simulink model "TestingDynamics"  (R2019b)
settings: Solver=VariableStepAuto  StartTime=0.0  StopTime=10.0  RelTol=1e-3
values from neighbouring files (symbols this model uses):
  M_inv = inv(M_motor)    [HW7_v2_matlab.m]
  M_motor = [1, 1, 1, -1;             1, 1, -1, 1;             1, -1, -1, -1;             1, -1, 1, 1 ]    [HW7_v2_matlab.m]
  measurement_noise = 0.1    [kalman_matrices_calculator.m]
  tau2 = eval(max(solve(1/sqrt((tau2*2*pi*10)^2+1^2) == 1/sqrt(2), tau2)))    [HW7_v2_matlab.m]    (also in kalman_matrices_calculator.m = 0.0159154943092)
  V = 5    [HW7_v2_matlab.m]
  V0 = 5    [HW7_v2_matlab.m]
undefined symbols (not defined in the file or in its folder): A, Aaileron, Aelevator, Arudder, Athrust, B, Baileron, Belevator, Brudder, Bthrust, C, C_P, C_rollpitch, C_T, C_yaw, Caileron, Celevator, Crudder, Cthrust, D, Daileron, Delevator, Drudder, Dthrust, g, J, Jinv, Prop_H, Thrust_Sum, trim_state, UAV_mass
libraries: vrlib x3, simulink x2, dspmtrx3 x1
settings Model: Creator=cwhipp  LastModifiedBy=cwhipp

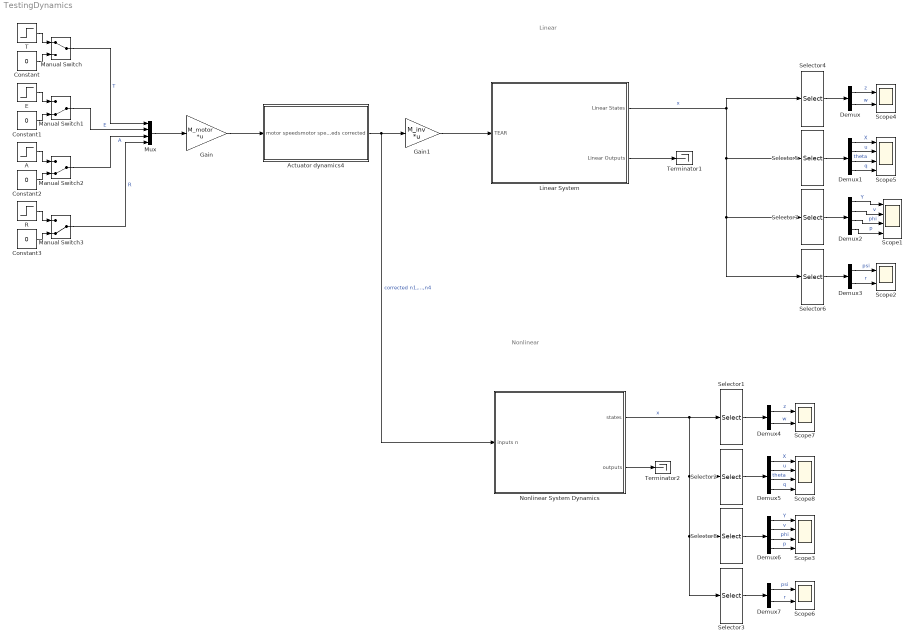
== system TestingDynamics ==
  note: Linear
  note: Nonlinear
  A : Step  SampleTime=0
  Actuator dynamics4 : Subsystem
  Constant{,1..3} (4 alike) : Constant  Value=0
  Demux{,3..4,7} (4 alike) : Demux  Outputs=2
  Demux{1..2,5..6} (4 alike) : Demux
  E : Step  SampleTime=0
  Gain : Gain  Gain=M_motor  Multiplication=Matrix(K*u)
  Gain1 : Gain  Gain=M_inv  Multiplication=Matrix(K*u)
  Linear System : Subsystem
  Manual Switch : ManualSwitch
  Manual Switch1 : ManualSwitch  CurrentSetting=0
  Manual Switch2 : ManualSwitch  CurrentSetting=0
  Manual Switch3 : ManualSwitch  CurrentSetting=0
  Mux : Mux
  Nonlinear System Dynamics : Subsystem
  R : Step  SampleTime=0
  Scope{1,3,5,8} (4 alike) : Scope  NumInputPorts=4
  Scope{2,4,6..7} (4 alike) : Scope  NumInputPorts=2
  Selector1 : Selector  InputPortWidth=12  IndexOptions=Index vector (dialog)  Indices=[3 6]  OutputSizes=1
  Selector2 : Selector  InputPortWidth=12  IndexOptions=Index vector (dialog)  Indices=[1 4 8 11]  OutputSizes=1
  Selector3 : Selector  InputPortWidth=12  IndexOptions=Index vector (dialog)  Indices=[9 12]  OutputSizes=1
  Selector4 : Selector  InputPortWidth=12  IndexOptions=Index vector (dialog)  Indices=[1 2]  OutputSizes=1
  Selector5 : Selector  InputPortWidth=12  IndexOptions=Index vector (dialog)  Indices=[3 4 5 6]  OutputSizes=1
  Selector6 : Selector  InputPortWidth=12  IndexOptions=Index vector (dialog)  Indices=[11 12]  OutputSizes=1
  Selector7 : Selector  InputPortWidth=12  IndexOptions=Index vector (dialog)  Indices=[7 8 9 10]  OutputSizes=1
  Selector8 : Selector  InputPortWidth=12  IndexOptions=Index vector (dialog)  Indices=[2 5 7 10]  OutputSizes=1
  T : Step  SampleTime=0
  Terminator1 : Terminator
  Terminator2 : Terminator
  wires:
  Linear System/1(Linear States) -> Selector4/1, Selector6/1, Selector7/1, Selector5/1  "x"
  Linear System/2(Linear Outputs) -> Terminator1/1
  Demux/2 -> Scope4/2  "w"
  Demux/1 -> Scope4/1  "z"
  Selector4/1 -> Demux/1
  Selector5/1 -> Demux1/1
  Demux1/1 -> Scope5/1  "X"
  Demux1/2 -> Scope5/2  "u"
  Demux1/3 -> Scope5/3  "theta"
  Demux1/4 -> Scope5/4  "q"
  T/1 -> Manual Switch/1
  Constant/1 -> Manual Switch/2
  E/1 -> Manual Switch1/1
  Constant1/1 -> Manual Switch1/2
  A/1 -> Manual Switch2/1
  Constant2/1 -> Manual Switch2/2
  R/1 -> Manual Switch3/1
  Constant3/1 -> Manual Switch3/2
  Manual Switch/1 -> Mux/1  "T"
  Manual Switch1/1 -> Mux/2  "E"
  Manual Switch2/1 -> Mux/3  "A"
  Manual Switch3/1 -> Mux/4  "R"
  Demux2/4 -> Scope1/4  "p"
  Demux2/1 -> Scope1/1  "Y"
  Selector7/1 -> Demux2/1
  Demux2/3 -> Scope1/3  "phi"
  Demux2/2 -> Scope1/2  "v"
  Demux3/2 -> Scope2/2  "r"
  Demux3/1 -> Scope2/1  "psi"
  Selector6/1 -> Demux3/1
  Gain/1 -> Actuator dynamics4/1(motor speeds)
  Mux/1 -> Gain/1
  Actuator dynamics4/1(motor speeds corrected) -> Nonlinear System Dynamics/1(inputs n), Gain1/1  "corrected n1,...,n4"
  Gain1/1 -> Linear System/1("TEAR ")
  Selector8/1 -> Demux6/1
  Demux7/2 -> Scope6/2  "r"
  Demux5/1 -> Scope8/1  "X"
  Nonlinear System Dynamics/1(states) -> Selector3/1, Selector8/1, Selector2/1, Selector1/1  "x"
  Demux5/4 -> Scope8/4  "q"
  Demux6/4 -> Scope3/4  "p"
  Selector1/1 -> Demux4/1
  Demux4/2 -> Scope7/2  "w"
  Demux4/1 -> Scope7/1  "z"
  Selector2/1 -> Demux5/1
  Demux6/1 -> Scope3/1  "Y"
  Demux6/3 -> Scope3/3  "phi"
  Selector3/1 -> Demux7/1
  Demux5/3 -> Scope8/3  "theta"
  Demux5/2 -> Scope8/2  "u"
  Demux7/1 -> Scope6/1  "psi"
  Demux6/2 -> Scope3/2  "v"
  Nonlinear System Dynamics/2(outputs) -> Terminator2/1

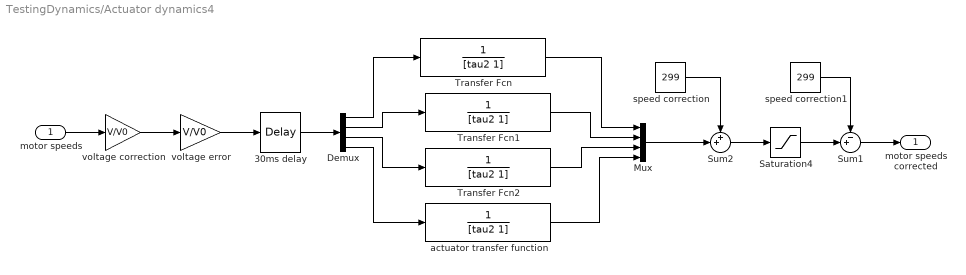
== system TestingDynamics/Actuator dynamics4 ==
  motor speeds : Inport
  30ms delay : TransportDelay  DelayTime=30e-3
  Demux : Demux
  Mux : Mux
  Saturation4 : Saturate  UpperLimit=500  LowerLimit=10
  Sum1 : Sum  Inputs=-+|
  Sum2 : Sum  Inputs=++|
  Transfer Fcn : TransferFcn  Denominator=[tau2 1]
  Transfer Fcn1 : TransferFcn  Denominator=[tau2 1]
  Transfer Fcn2 : TransferFcn  Denominator=[tau2 1]
  actuator transfer function : TransferFcn  Denominator=[tau2 1]
  speed correction : Constant  Value=299
  speed correction1 : Constant  Value=299
  voltage correction : Gain  Gain=V/V0
  voltage error : Gain  Gain=V/V0
  motor speeds corrected : Outport
  wires:
  speed correction/1 -> Sum2/1
  voltage correction/1 -> voltage error/1
  Sum2/1 -> Saturation4/1
  Demux/2 -> Transfer Fcn1/1
  30ms delay/1 -> Demux/1
  Demux/4 -> actuator transfer function/1
  Demux/1 -> Transfer Fcn/1
  Demux/3 -> Transfer Fcn2/1
  voltage error/1 -> 30ms delay/1
  motor speeds/1 -> voltage correction/1
  Transfer Fcn/1 -> Mux/1
  Transfer Fcn1/1 -> Mux/2
  Transfer Fcn2/1 -> Mux/3
  actuator transfer function/1 -> Mux/4
  Mux/1 -> Sum2/2
  Saturation4/1 -> Sum1/2
  Sum1/1 -> motor speeds corrected/1
  speed correction1/1 -> Sum1/1

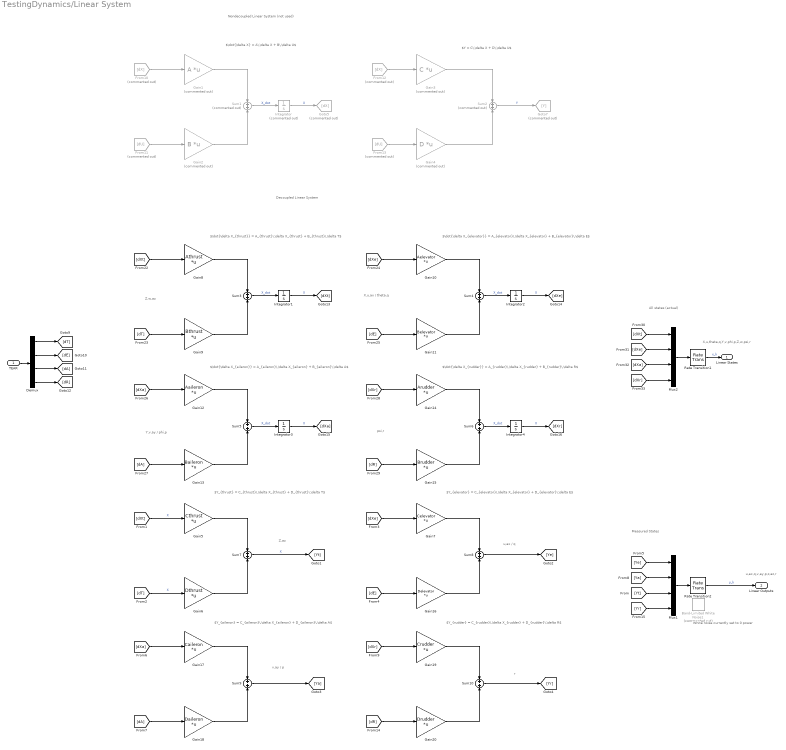
== system TestingDynamics/Linear System ==
  note: psi,r
  note: Y,v,ay / phi,p
  note: X,u,ax / theta,q
  note: Z,w,az
  note: Decoupled Linear System
  note: $\dot{\delta X} = A\,\delta X + B\,\delta U$
  note: $Y = C\,\delta X + D\,\delta U$
  note: $\dot{\delta X_{thrust}} = A_{thrust}\,\delta X_{thrust} + B_{thrust}\,\delta T$
  note: $\dot{\delta X_{elevator}} = A_{elevator}\,\delta X_{elevator} + B_{elevator}\,\delta E$
  note: $\dot{\delta X_{aileron}} = A_{aileron}\,\delta X_{aileron} + B_{aileron}\,\delta A$
  note: $\dot{\delta X_{rudder}} = A_{rudder}\,\delta X_{rudder} + B_{rudder}\,\delta R$
  note: Z,az
  note: u,ax / q
  note: v,ay / p
  note: r
  note: $Y_{thrust} = C_{thrust}\,\delta X_{thrust} + D_{thrust}\,\delta T$
  note: $Y_{elevator} = C_{elevator}\,\delta X_{elevator} + D_{elevator}\,\delta E$
  note: $Y_{aileron} = C_{aileron}\,\delta X_{aileron} + D_{aileron}\,\delta A$
  note: $Y_{rudder} = C_{rudder}\,\delta X_{rudder} + D_{rudder}\,\delta R$
  note: Nondecoupled Linear System (not used)
  note: All states (actual)
  note: Measured States
  note: u,ax,q,v,ay,p,z,az,r
  note: X,u,theta,q,Y,v,phi,p,Z,w,psi,r
  note: White noise currently set to 0 power
  "TEAR " : Inport
  Band-Limited White Noise1 : simulink/Sources/Band-Limited White Noise  Commented=on  Cov=measurement_noise*ones(9,1)*0  Ts=0.05  seed=[11;12;13;14;15;16;17;18;19]
  Demux : Demux
  From10 : From  Commented=on  GotoTag=dX
  From11 : From  Commented=on  GotoTag=dU
  From12 : From  Commented=on  GotoTag=dX
  From13 : From  Commented=on  GotoTag=dU
  Gain1 : Gain  Commented=on  Gain=A  Multiplication=Matrix(K*u)
  Gain10 : Gain  Gain=Aelevator  Multiplication=Matrix(K*u)
  Gain11 : Gain  Gain=Belevator  Multiplication=Matrix(K*u)
  Gain12 : Gain  Gain=Aaileron  Multiplication=Matrix(K*u)
  Gain13 : Gain  Gain=Baileron  Multiplication=Matrix(K*u)
  Gain14 : Gain  Gain=Arudder  Multiplication=Matrix(K*u)
  Gain15 : Gain  Gain=Brudder  Multiplication=Matrix(K*u)
  Gain16 : Gain  Gain=Delevator  Multiplication=Matrix(K*u)
  Gain17 : Gain  Gain=Caileron  Multiplication=Matrix(K*u)
  Gain18 : Gain  Gain=Daileron  Multiplication=Matrix(K*u)
  Gain19 : Gain  Gain=Crudder  Multiplication=Matrix(K*u)
  Gain2 : Gain  Commented=on  Gain=B  Multiplication=Matrix(K*u)
  Gain20 : Gain  Gain=Drudder  Multiplication=Matrix(K*u)
  Gain3 : Gain  Commented=on  Gain=C  Multiplication=Matrix(K*u)
  Gain4 : Gain  Commented=on  Gain=D  Multiplication=Matrix(K*u)
  Gain5 : Gain  Gain=Cthrust  Multiplication=Matrix(K*u)
  Gain6 : Gain  Gain=Dthrust  Multiplication=Matrix(K*u)
  Gain7 : Gain  Gain=Celevator  Multiplication=Matrix(K*u)
  Gain8 : Gain  Gain=Athrust  Multiplication=Matrix(K*u)
  Gain9 : Gain  Gain=Bthrust  Multiplication=Matrix(K*u)
  Goto5 : Goto  Commented=on  GotoTag=dX
  Goto7 : Goto  Commented=on  GotoTag=Y
  Integrator : Integrator  Commented=on  InitialCondition=trim_state
  Integrator1 : Integrator  InitialCondition=trim_state(9:10)
  Integrator2 : Integrator  InitialCondition=trim_state(1:4)
  Integrator3 : Integrator  InitialCondition=trim_state(5:8)
  Integrator4 : Integrator  InitialCondition=trim_state(11:12)
  Mux1 : Mux
  Mux2 : Mux
  Rate Transition1 : RateTransition  OutPortSampleTime=0.005
  Rate Transition2 : RateTransition  OutPortSampleTime=0.005
  Sum1 : Sum  Commented=on  Inputs=+|+
  Sum{3..10} (8 alike) : Sum  Inputs=+|+
  Sum2 : Sum  Commented=on  Inputs=+|+
  Linear States : Outport
  Linear Outputs : Outport  Port=2
  wires:
  Gain14/1 -> Sum6/1
  From11/1 -> Gain2/1
  [dXe] -> Gain10/1
  Gain10/1 -> Sum4/1
  Gain2/1 -> Sum1/2
  Gain15/1 -> Sum6/2
  Gain1/1 -> Sum1/1
  Sum5/1 -> Integrator3/1  "X_dot"
  Gain3/1 -> Sum2/1
  Integrator1/1 -> [dXt]  "X"
  From10/1 -> Gain1/1
  Sum1/1 -> Integrator/1  "X_dot"
  Sum2/1 -> Goto7/1  "Y"
  Integrator3/1 -> [dXa]  "X"
  Gain8/1 -> Sum3/1
  [dXt] -> Gain8/1
  Sum3/1 -> Integrator1/1  "X_dot"
  Integrator4/1 -> [dXr]  "X"
  Sum4/1 -> Integrator2/1  "X_dot"
  Gain13/1 -> Sum5/2
  [dXa] -> Gain12/1
  [dXr] -> Gain14/1
  Sum6/1 -> Integrator4/1  "X_dot"
  From13/1 -> Gain4/1
  Gain11/1 -> Sum4/2
  Integrator/1 -> Goto5/1  "X"
  Gain4/1 -> Sum2/2
  Gain12/1 -> Sum5/1
  Integrator2/1 -> [dXe]  "X"
  From12/1 -> Gain3/1
  "TEAR "/1 -> Demux/1
  Demux/3 -> [dA]
  Demux/2 -> [dE]
  Demux/1 -> [dT]
  Demux/4 -> [dR]
  [dXa] -> Mux2/3
  [dXr] -> Mux2/4
  Mux2/1 -> Rate Transition1/1
  [dXt] -> Mux2/1
  [dXe] -> Mux2/2
  Gain6/1 -> Sum7/2
  Gain5/1 -> Sum7/1
  Gain16/1 -> Sum8/2
  [dE] -> Gain16/1
  Gain7/1 -> Sum8/1
  [dXe] -> Gain7/1
  [dA] -> Gain18/1
  Gain17/1 -> Sum9/1
  [dXa] -> Gain17/1
  Gain18/1 -> Sum9/2
  [dXr] -> Gain19/1
  [dR] -> Gain20/1
  Gain20/1 -> Sum10/2
  Gain19/1 -> Sum10/1
  [Ya] -> Mux1/2
  [Ye] -> Mux1/1
  Mux1/1 -> Rate Transition2/1
  [Yr] -> Mux1/4
  [Yt] -> Mux1/3
  [dT] -> Gain9/1
  [dA] -> Gain13/1
  [dR] -> Gain15/1
  [dE] -> Gain11/1
  Sum9/1 -> [Ya]
  Sum10/1 -> [Yr]
  Sum8/1 -> [Ye]
  Gain9/1 -> Sum3/2
  [dT] -> Gain6/1  "X"
  [dXt] -> Gain5/1  "X"
  Sum7/1 -> [Yt]  "X"
  Rate Transition1/1 -> Linear States/1  "x_k"
  Rate Transition2/1 -> Linear Outputs/1  "y_k"

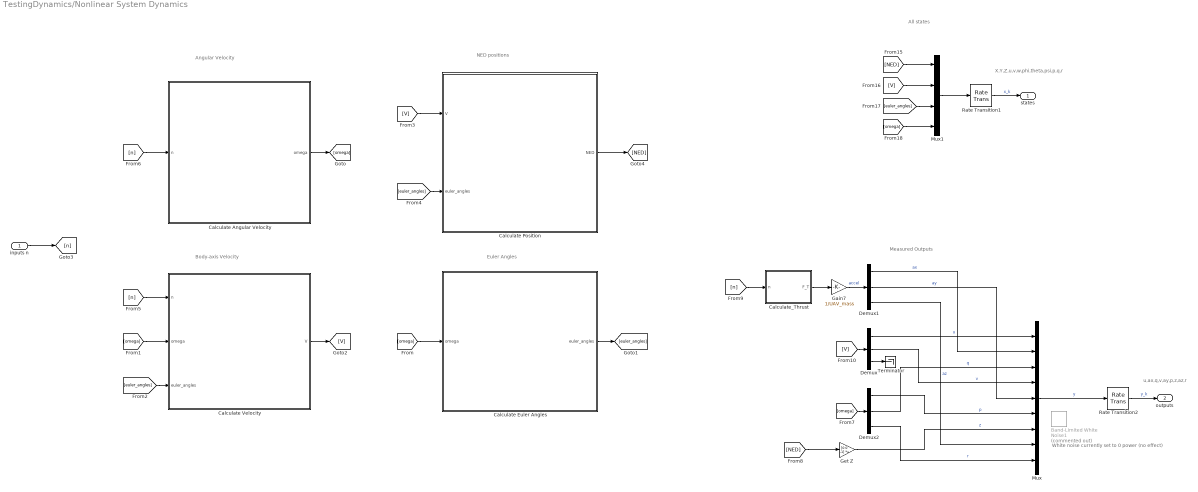
== system TestingDynamics/Nonlinear System Dynamics ==
  note: White noise currently set to 0 power (no effect)
  note: X,Y,Z,u,v,w,phi,theta,psi,p,q,r
  note: Euler Angles
  note: NED positions
  note: Angular Velocity
  note: Body-axis Velocity
  note: u,ax,q,v,ay,p,z,az,r
  note: All states
  note: Measured Outputs
  inputs n : Inport
  Band-Limited White Noise1 : simulink/Sources/Band-Limited White Noise  Commented=on  Cov=measurement_noise*ones(9,1)*0  Ts=0.05  seed=[11;12;13;14;15;16;17;18;19]
  Calculate Angular Velocity : Subsystem
  Calculate Euler Angles : Subsystem
  Calculate Position : Subsystem
  Calculate Velocity : Subsystem
  Calculate_Thrust : Subsystem
  Demux : Demux  Outputs=3
  Demux1 : Demux  Outputs=3
  Demux2 : Demux  Outputs=3
  Gain7 : Gain  Gain=1/UAV_mass
      settings: AttributesFormatString=%<Gain>
  Get Z : Gain  Gain=[0 0 -1]  Multiplication=Matrix(K*u)
  Mux : Mux  Inputs=9
  Mux1 : Mux
  Rate Transition1 : RateTransition  OutPortSampleTime=0.005
  Rate Transition2 : RateTransition  OutPortSampleTime=0.005
  Terminator : Terminator
  states : Outport
  outputs : Outport  Port=2
  wires:
  [euler_angles] -> Mux1/3
  [omega] -> Mux1/4
  Calculate Euler Angles/1(euler_angles) -> [euler_angles]
  [V] -> Calculate Position/1("V ")
  [euler_angles] -> Calculate Position/2(euler_angles)
  Calculate Angular Velocity/1(omega) -> [omega]
  [omega] -> Calculate Euler Angles/1(omega)
  Calculate Velocity/1(V) -> [V]
  [V] -> Mux1/2
  [NED] -> Mux1/1
  [euler_angles] -> Calculate Velocity/3(euler_angles)
  [omega] -> Calculate Velocity/2(omega)
  [n] -> Calculate Velocity/1(n)
  Calculate Position/1(NED) -> [NED]
  [n] -> Calculate Angular Velocity/1(n)
  Mux1/1 -> Rate Transition1/1
  inputs n/1 -> [n]
  Demux1/1 -> Mux/2  "ax"
  Demux/1 -> Mux/1  "u"
  Mux/1 -> Rate Transition2/1  "y"
  Demux/3 -> Terminator/1
  [omega] -> Demux2/1
  [NED] -> Get Z/1
  Get Z/1 -> Mux/7  "z"
  Demux2/2 -> Mux/3  "q"
  Demux/2 -> Mux/4  "v"
  Demux2/1 -> Mux/6  "p"
  Demux1/2 -> Mux/5  "ay"
  Demux2/3 -> Mux/9  "r"
  [V] -> Demux/1
  Demux1/3 -> Mux/8  "az"
  Gain7/1 -> Demux1/1  "accel"
  Calculate_Thrust/1(F_T) -> Gain7/1
  [n] -> Calculate_Thrust/1(n)
  Rate Transition1/1 -> states/1  "x_k"
  Rate Transition2/1 -> outputs/1  "y_k"

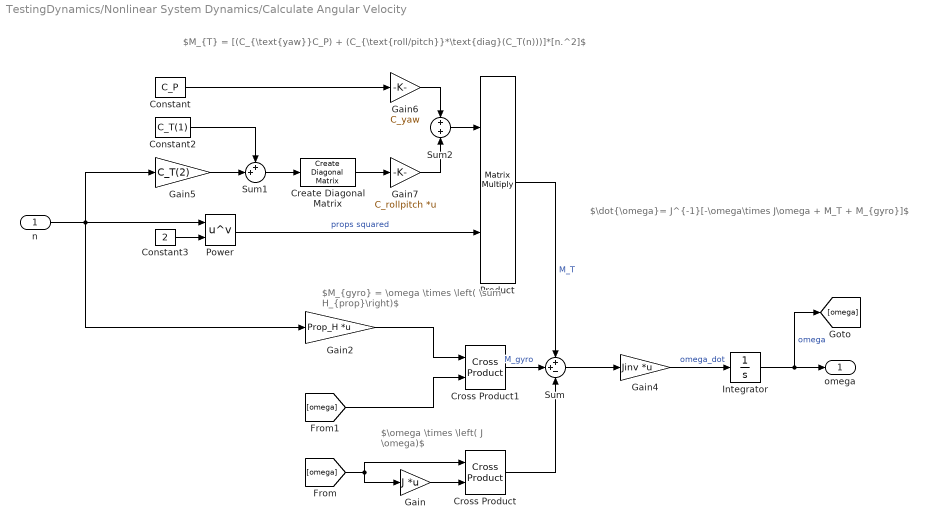
== system TestingDynamics/Nonlinear System Dynamics/Calculate Angular Velocity ==
  note: $M_{gyro} = \omega \times \left( \sum H_{prop}\right)$
  note: $\dot{\omega}= J^{-1}[-\omega\times J\omega + M_T + M_{gyro}]$
  note: $\omega \times \left( J \omega)$
  note: $M_{T} = [(C_{\text{yaw}}C_P) + (C_{\text{roll/pitch}}*\text{diag}(C_T(n)))]*[n.^2]$
  n : Inport
  Constant : Constant  Value=C_P
  Constant2 : Constant  Value=C_T(1)
  Constant3 : Constant  Value=2
  Create Diagonal Matrix : dspmtrx3/Create Diagonal Matrix
      settings: SourceProductName=DSP System Toolbox  SourceProductBaseCode=DS
  Cross Product : vrlib/Utilities/Cross Product
      settings: SourceProductName=Simulink
  Cross Product1 : vrlib/Utilities/Cross Product
      settings: SourceProductName=Simulink
  Gain : Gain  Gain=J  Multiplication=Matrix(K*u)
  Gain2 : Gain  Gain=Prop_H  Multiplication=Matrix(K*u)
  Gain4 : Gain  Gain=Jinv  Multiplication=Matrix(K*u)
      settings: AttributesFormatString=%<Gain>
  Gain5 : Gain  Gain=C_T(2)
  Gain6 : Gain  Gain=C_yaw
      settings: AttributesFormatString=%<Gain>
  Gain7 : Gain  Gain=C_rollpitch  Multiplication=Matrix(K*u)
      settings: AttributesFormatString=%<Gain>
  Integrator : Integrator  InitialCondition=[0;0;0]
  Power : Math  Operator=pow  SignedPower=off  SaturateOnIntegerOverflow=on
  Product : Product  Multiplication=Matrix(*)
  Sum : Sum  Inputs=++-
  Sum1 : Sum  Inputs=++|
  Sum2 : Sum  Inputs=+|+
  omega : Outport
  wires:
  Sum/1 -> Gain4/1
  [omega] -> Gain/1, Cross Product/1
  Cross Product/1 -> Sum/3
  [omega] -> Cross Product1/2
  Gain2/1 -> Cross Product1/1
  Cross Product1/1 -> Sum/2  "M_gyro"
  Gain4/1 -> Integrator/1  "omega_dot"
  Gain/1 -> Cross Product/2
  Integrator/1 -> [omega], omega/1  "omega"
  Product/1 -> Sum/1  "M_T"
  Create Diagonal Matrix/1 -> Gain7/1
  Sum2/1 -> Product/1
  Sum1/1 -> Create Diagonal Matrix/1
  Constant/1 -> Gain6/1
  Power/1 -> Product/2  "props squared"
  Gain6/1 -> Sum2/1
  Gain5/1 -> Sum1/2
  Gain7/1 -> Sum2/2
  n/1 -> Gain2/1, Power/1, Gain5/1
  Constant2/1 -> Sum1/1
  Constant3/1 -> Power/2

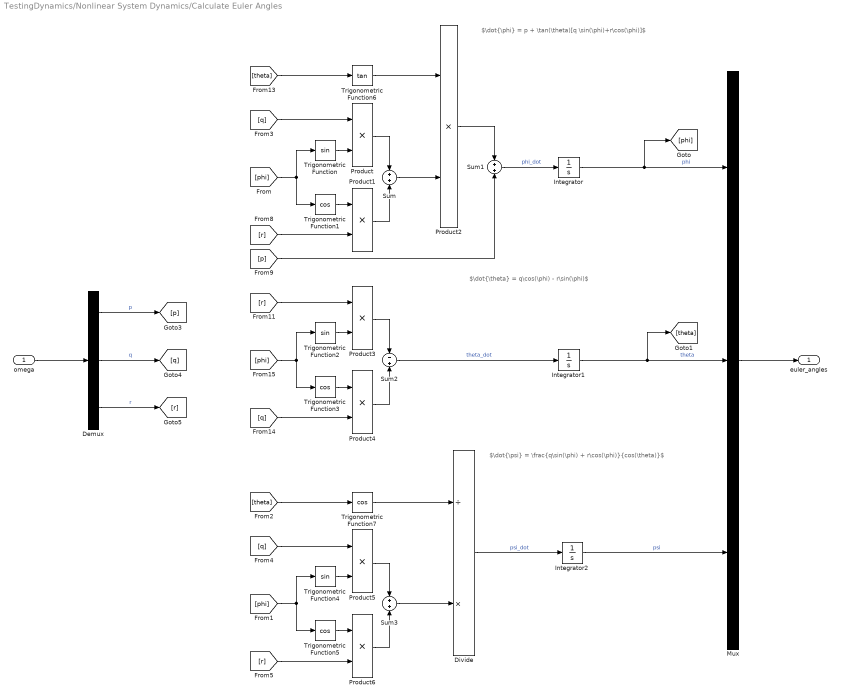
== system TestingDynamics/Nonlinear System Dynamics/Calculate Euler Angles ==
  note: $\dot{\phi} = p + \tan(\theta)[q \sin(\phi)+r\cos(\phi)]$
  note: $\dot{\theta} = q\cos(\phi) - r\sin(\phi)$
  note: $\dot{\psi} = \frac{q\sin(\phi) + r\cos(\phi)}{cos(\theta)}$
  omega : Inport
  Demux : Demux  Outputs=3
  Divide : Product  Inputs=/*
  Integrator : Integrator
  Integrator1 : Integrator
  Integrator2 : Integrator
  Mux : Mux  Inputs=3
  Product{,1..6} (7 alike) : Product
  Sum : Sum  Inputs=+|+
  Sum1 : Sum  Inputs=+|+
  Sum2 : Sum  Inputs=-|+
  Sum3 : Sum  Inputs=+|+
  Trigonometric Function : Trigonometry
  Trigonometric Function{1,3,5,7} (4 alike) : Trigonometry  Operator=cos
  Trigonometric Function2 : Trigonometry
  Trigonometric Function4 : Trigonometry
  Trigonometric Function6 : Trigonometry  Operator=tan
  euler_angles : Outport
  wires:
  Trigonometric Function7/1 -> Divide/1
  Product1/1 -> Sum/2
  Product6/1 -> Sum3/2
  Trigonometric Function/1 -> Product/2
  Product5/1 -> Sum3/1
  [theta] -> Trigonometric Function7/1
  Trigonometric Function6/1 -> Product2/1
  [r] -> Product6/2
  [theta] -> Trigonometric Function6/1
  Integrator1/1 -> [theta], Mux/2  "theta"
  Trigonometric Function4/1 -> Product5/2
  [q] -> Product4/2
  Demux/3 -> [r]  "r"
  Divide/1 -> Integrator2/1  "psi_dot"
  Integrator2/1 -> Mux/3  "psi"
  [q] -> Product5/1
  Product4/1 -> Sum2/2
  [q] -> Product/1
  [phi] -> Trigonometric Function4/1, Trigonometric Function5/1
  Sum2/1 -> Integrator1/1  "theta_dot"
  Trigonometric Function5/1 -> Product6/1
  Trigonometric Function3/1 -> Product4/1
  [r] -> Product3/1
  Integrator/1 -> [phi], Mux/1  "phi"
  Sum3/1 -> Divide/2
  Product3/1 -> Sum2/1
  [phi] -> Trigonometric Function2/1, Trigonometric Function3/1
  Demux/1 -> [p]  "p"
  Product2/1 -> Sum1/1
  [r] -> Product1/2
  Trigonometric Function1/1 -> Product1/1
  [phi] -> Trigonometric Function1/1, Trigonometric Function/1
  omega/1 -> Demux/1
  Product/1 -> Sum/1
  Demux/2 -> [q]  "q"
  Sum/1 -> Product2/2
  Mux/1 -> euler_angles/1
  Sum1/1 -> Integrator/1  "phi_dot"
  [p] -> Sum1/2
  Trigonometric Function2/1 -> Product3/2

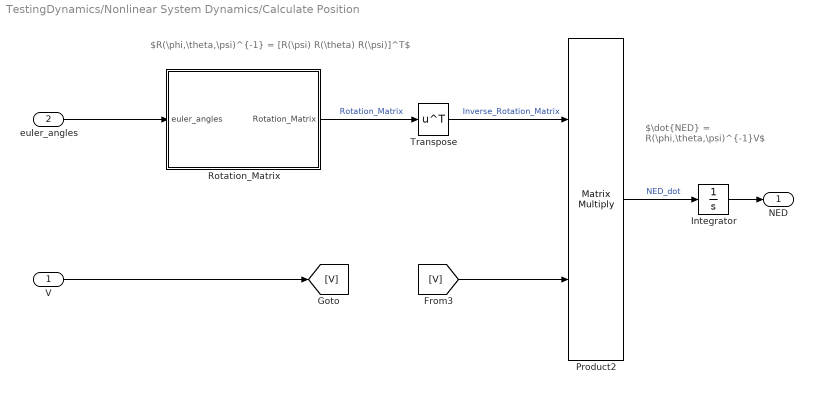
== system TestingDynamics/Nonlinear System Dynamics/Calculate Position ==
  note: $R(\phi,\theta,\psi)^{-1} = [R(\psi) R(\theta) R(\psi)]^T$
  note: $\dot{NED} = R(\phi,\theta,\psi)^{-1}V$
  "V " : Inport
  euler_angles : Inport  Port=2
  Integrator : Integrator  InitialCondition=[0;0;0]
  Product2 : Product  Multiplication=Matrix(*)
  Rotation_Matrix : Subsystem
  Transpose : Math  Operator=transpose  SignedPower=off  SaturateOnIntegerOverflow=on
  NED : Outport
  wires:
  Product2/1 -> Integrator/1  "NED_dot"
  "V "/1 -> [V]
  Rotation_Matrix/1(Rotation_Matrix) -> Transpose/1  "Rotation_Matrix"
  Transpose/1 -> Product2/1  "Inverse_Rotation_Matrix"
  [V] -> Product2/2
  euler_angles/1 -> Rotation_Matrix/1("euler_angles ")
  Integrator/1 -> NED/1

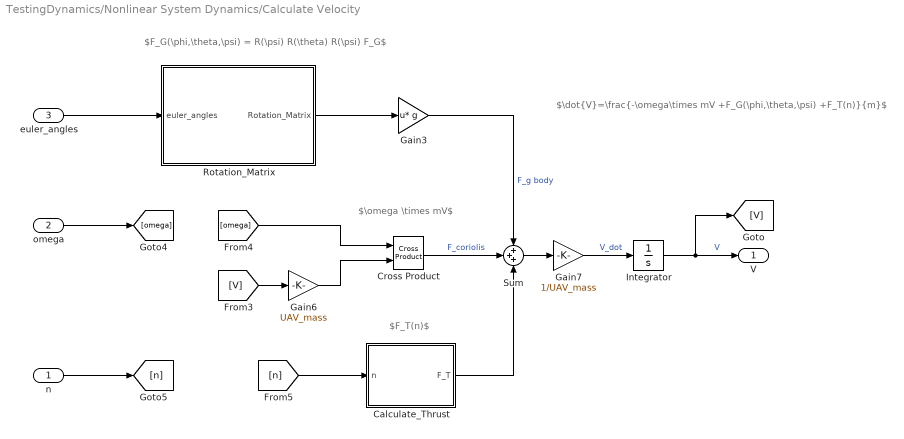
== system TestingDynamics/Nonlinear System Dynamics/Calculate Velocity ==
  note: $F_G(\phi,\theta,\psi) = R(\psi) R(\theta) R(\psi) F_G$
  note: $\dot{V}=\frac{-\omega\times mV +F_G(\phi,\theta,\psi) +F_T(n)}{m}$
  note: $\omega \times mV$
  note: $F_T(n)$
  n : Inport
  omega : Inport  Port=2
  euler_angles : Inport  Port=3
  Calculate_Thrust : Subsystem
  Cross Product : vrlib/Utilities/Cross Product
      settings: SourceProductName=Simulink
  Gain3 : Gain  Gain=g  Multiplication=Matrix(u*K)
      settings: AttributesFormatString=%<Gain>
  Gain6 : Gain  Gain=UAV_mass
      settings: AttributesFormatString=%<Gain>
  Gain7 : Gain  Gain=1/UAV_mass
      settings: AttributesFormatString=%<Gain>
  Integrator : Integrator  InitialCondition=[0;0;0]
  Rotation_Matrix : Subsystem
  Sum : Sum  Inputs=+++
  V : Outport
  wires:
  [V] -> Gain6/1
  [omega] -> Cross Product/1
  Cross Product/1 -> Sum/2  "F_coriolis"
  Gain3/1 -> Sum/1  "F_g body"
  Gain6/1 -> Cross Product/2
  Sum/1 -> Gain7/1
  Integrator/1 -> V/1, [V]  "V"
  omega/1 -> [omega]
  n/1 -> [n]
  Rotation_Matrix/1(Rotation_Matrix) -> Gain3/1
  euler_angles/1 -> Rotation_Matrix/1("euler_angles ")
  [n] -> Calculate_Thrust/1(n)
  Gain7/1 -> Integrator/1  "V_dot"
  Calculate_Thrust/1(F_T) -> Sum/3

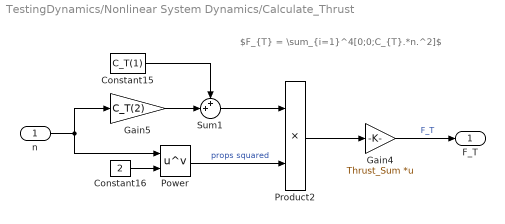
== system TestingDynamics/Nonlinear System Dynamics/Calculate_Thrust ==
  note: $F_{T} = \sum_{i=1}^4[0;0;C_{T}.*n.^2]$
  n : Inport
  Constant15 : Constant  Value=C_T(1)
  Constant16 : Constant  Value=2
  Gain4 : Gain  Gain=Thrust_Sum  Multiplication=Matrix(K*u)
      settings: AttributesFormatString=%<Gain>
  Gain5 : Gain  Gain=C_T(2)
  Power : Math  Operator=pow  SignedPower=off  SaturateOnIntegerOverflow=on
  Product2 : Product
  Sum1 : Sum  Inputs=++|
  F_T : Outport
  wires:
  Constant15/1 -> Sum1/1
  Gain4/1 -> F_T/1  "F_T"
  n/1 -> Power/1, Gain5/1
  Power/1 -> Product2/2  "props squared"
  Gain5/1 -> Sum1/2
  Sum1/1 -> Product2/1
  Product2/1 -> Gain4/1
  Constant16/1 -> Power/2

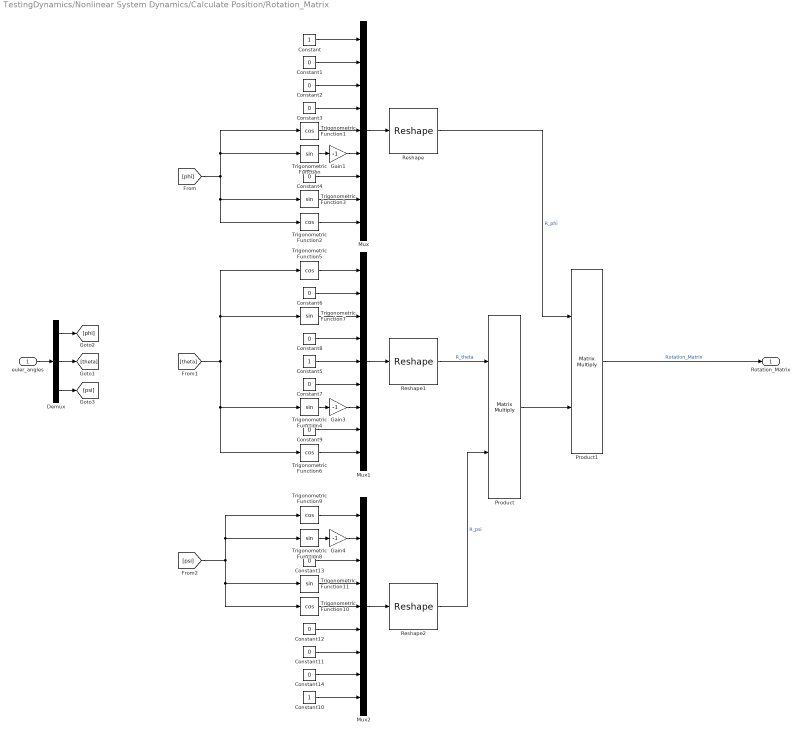
== system TestingDynamics/Nonlinear System Dynamics/Calculate Position/Rotation_Matrix ==
  "euler_angles " : Inport
  Constant : Constant
  Constant{1..4,6..9,11..14} (12 alike) : Constant  Value=0
  Constant10 : Constant
  Constant5 : Constant
  Demux : Demux  Outputs=3
  Gain1 : Gain  Gain=-1
  Gain3 : Gain  Gain=-1
  Gain4 : Gain  Gain=-1
  Mux : Mux  Inputs=9
  Mux1 : Mux  Inputs=9
  Mux2 : Mux  Inputs=9
  Product : Product  Multiplication=Matrix(*)
  Product1 : Product  Multiplication=Matrix(*)
  Reshape : Reshape  OutputDimensionality=Customize  OutputDimensions=[3,3]
  Reshape1 : Reshape  OutputDimensionality=Customize  OutputDimensions=[3,3]
  Reshape2 : Reshape  OutputDimensionality=Customize  OutputDimensions=[3,3]
  Trigonometric Function{,3..4,7..8,11} (6 alike) : Trigonometry
  Trigonometric Function{1..2,5..6,9..10} (6 alike) : Trigonometry  Operator=cos
  Rotation_Matrix : Outport
  wires:
  Constant9/1 -> Mux1/8
  Constant11/1 -> Mux2/7
  Trigonometric Function1/1 -> Mux/5
  Trigonometric Function3/1 -> Mux/8
  Constant5/1 -> Mux1/5
  Trigonometric Function7/1 -> Mux1/3
  Reshape/1 -> Product1/1  "R_phi"
  Mux1/1 -> Reshape1/1
  Trigonometric Function8/1 -> Gain4/1
  Constant7/1 -> Mux1/6
  Trigonometric Function2/1 -> Mux/9
  [phi] -> Trigonometric Function2/1, Trigonometric Function3/1, Trigonometric Function1/1, Trigonometric Function/1
  Trigonometric Function6/1 -> Mux1/9
  Constant12/1 -> Mux2/6
  Trigonometric Function4/1 -> Gain3/1
  [theta] -> Trigonometric Function7/1, Trigonometric Function5/1, Trigonometric Function4/1, Trigonometric Function6/1
  Reshape2/1 -> Product/2  "R_psi"
  Trigonometric Function/1 -> Gain1/1
  Product/1 -> Product1/2
  Trigonometric Function5/1 -> Mux1/1
  Trigonometric Function9/1 -> Mux2/1
  Mux/1 -> Reshape/1
  Constant/1 -> Mux/1
  Constant3/1 -> Mux/4
  Constant6/1 -> Mux1/2
  Mux2/1 -> Reshape2/1
  Constant2/1 -> Mux/3
  Constant1/1 -> Mux/2
  [psi] -> Trigonometric Function11/1, Trigonometric Function10/1, Trigonometric Function9/1, Trigonometric Function8/1
  Constant8/1 -> Mux1/4
  Constant4/1 -> Mux/7
  Constant13/1 -> Mux2/3
  Trigonometric Function11/1 -> Mux2/4
  Constant10/1 -> Mux2/9
  Reshape1/1 -> Product/1  "R_theta"
  Constant14/1 -> Mux2/8
  Trigonometric Function10/1 -> Mux2/5
  Product1/1 -> Rotation_Matrix/1  "Rotation_Matrix"
  Demux/3 -> [psi]
  Demux/2 -> [theta]
  "euler_angles "/1 -> Demux/1
  Demux/1 -> [phi]
  Gain3/1 -> Mux1/7
  Gain1/1 -> Mux/6
  Gain4/1 -> Mux2/2

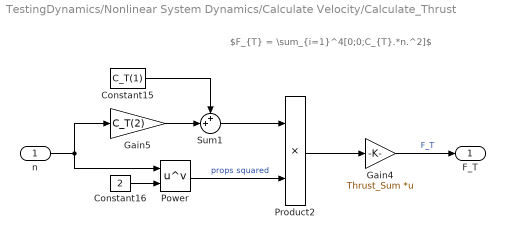
== system TestingDynamics/Nonlinear System Dynamics/Calculate Velocity/Calculate_Thrust ==
  note: $F_{T} = \sum_{i=1}^4[0;0;C_{T}.*n.^2]$
  n : Inport
  Constant15 : Constant  Value=C_T(1)
  Constant16 : Constant  Value=2
  Gain4 : Gain  Gain=Thrust_Sum  Multiplication=Matrix(K*u)
      settings: AttributesFormatString=%<Gain>
  Gain5 : Gain  Gain=C_T(2)
  Power : Math  Operator=pow  SignedPower=off  SaturateOnIntegerOverflow=on
  Product2 : Product
  Sum1 : Sum  Inputs=++|
  F_T : Outport
  wires:
  Constant15/1 -> Sum1/1
  Gain4/1 -> F_T/1  "F_T"
  n/1 -> Power/1, Gain5/1
  Power/1 -> Product2/2  "props squared"
  Gain5/1 -> Sum1/2
  Sum1/1 -> Product2/1
  Product2/1 -> Gain4/1
  Constant16/1 -> Power/2

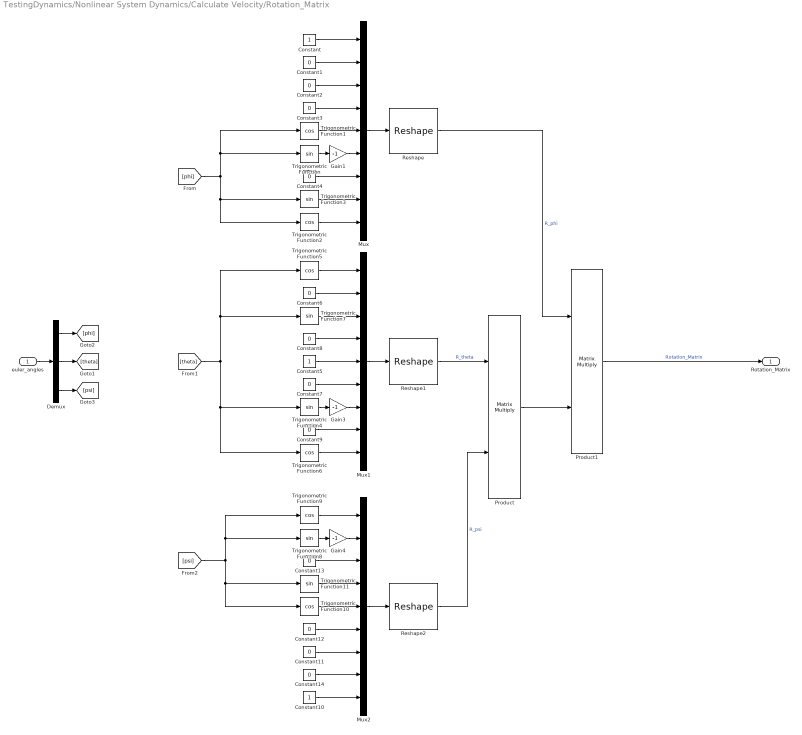
== system TestingDynamics/Nonlinear System Dynamics/Calculate Velocity/Rotation_Matrix ==
  "euler_angles " : Inport
  Constant : Constant
  Constant{1..4,6..9,11..14} (12 alike) : Constant  Value=0
  Constant10 : Constant
  Constant5 : Constant
  Demux : Demux  Outputs=3
  Gain1 : Gain  Gain=-1
  Gain3 : Gain  Gain=-1
  Gain4 : Gain  Gain=-1
  Mux : Mux  Inputs=9
  Mux1 : Mux  Inputs=9
  Mux2 : Mux  Inputs=9
  Product : Product  Multiplication=Matrix(*)
  Product1 : Product  Multiplication=Matrix(*)
  Reshape : Reshape  OutputDimensionality=Customize  OutputDimensions=[3,3]
  Reshape1 : Reshape  OutputDimensionality=Customize  OutputDimensions=[3,3]
  Reshape2 : Reshape  OutputDimensionality=Customize  OutputDimensions=[3,3]
  Trigonometric Function{,3..4,7..8,11} (6 alike) : Trigonometry
  Trigonometric Function{1..2,5..6,9..10} (6 alike) : Trigonometry  Operator=cos
  Rotation_Matrix : Outport
  wires:
  Constant9/1 -> Mux1/8
  Constant11/1 -> Mux2/7
  Trigonometric Function1/1 -> Mux/5
  Trigonometric Function3/1 -> Mux/8
  Constant5/1 -> Mux1/5
  Trigonometric Function7/1 -> Mux1/3
  Reshape/1 -> Product1/1  "R_phi"
  Mux1/1 -> Reshape1/1
  Trigonometric Function8/1 -> Gain4/1
  Constant7/1 -> Mux1/6
  Trigonometric Function2/1 -> Mux/9
  [phi] -> Trigonometric Function2/1, Trigonometric Function3/1, Trigonometric Function1/1, Trigonometric Function/1
  Trigonometric Function6/1 -> Mux1/9
  Constant12/1 -> Mux2/6
  Trigonometric Function4/1 -> Gain3/1
  [theta] -> Trigonometric Function7/1, Trigonometric Function5/1, Trigonometric Function4/1, Trigonometric Function6/1
  Reshape2/1 -> Product/2  "R_psi"
  Trigonometric Function/1 -> Gain1/1
  Product/1 -> Product1/2
  Trigonometric Function5/1 -> Mux1/1
  Trigonometric Function9/1 -> Mux2/1
  Mux/1 -> Reshape/1
  Constant/1 -> Mux/1
  Constant3/1 -> Mux/4
  Constant6/1 -> Mux1/2
  Mux2/1 -> Reshape2/1
  Constant2/1 -> Mux/3
  Constant1/1 -> Mux/2
  [psi] -> Trigonometric Function11/1, Trigonometric Function10/1, Trigonometric Function9/1, Trigonometric Function8/1
  Constant8/1 -> Mux1/4
  Constant4/1 -> Mux/7
  Constant13/1 -> Mux2/3
  Trigonometric Function11/1 -> Mux2/4
  Constant10/1 -> Mux2/9
  Reshape1/1 -> Product/1  "R_theta"
  Constant14/1 -> Mux2/8
  Trigonometric Function10/1 -> Mux2/5
  Product1/1 -> Rotation_Matrix/1  "Rotation_Matrix"
  Demux/3 -> [psi]
  Demux/2 -> [theta]
  "euler_angles "/1 -> Demux/1
  Demux/1 -> [phi]
  Gain3/1 -> Mux1/7
  Gain1/1 -> Mux/6
  Gain4/1 -> Mux2/2
